simulink model "Syr_ctrl_SFun"  (R2019b)
settings: Solver=ode3  StartTime=0.0  StopTime=0.3  FixedStep=Tstep  MaxStep=1e-5  RelTol=1e-3  AbsTol=1e-3  EnableMultiTasking=on
InitFcn:
  | tic
  | init_sim
  | mex Syr_ctrl.c User_functions\Src\*.c
StopFcn:
  | elapsed_time=toc
values from neighbouring files (symbols this model uses):
  accel = 1000    [init_sim.m]
  B = 0    [init_sim.m]
  Ctrl_type = 3    [init_sim.m]
  dT = motorModel.SyreDrive.Converter.dT    [init_sim.m]
  Fd = motorModel.idiq.Fd    [init_sim.m]
  Fd_dqt = motorModel.dqtMapF.dataF.Fd    [init_sim.m]
  Fd_max = max(Fd_dqt,[],'all')    [init_sim.m]
  Fd_min = min(Fd_dqt,[],'all')    [init_sim.m]
  FMapsModel = -1    [init_sim.m]
  Fq = motorModel.idiq.Fq    [init_sim.m]
  Fq_dqt = motorModel.dqtMapF.dataF.Fq    [init_sim.m]
  Fq_max = max(Fq_dqt,[],'all')    [init_sim.m]
  Fq_min = min(Fq_dqt,[],'all')    [init_sim.m]
  Id_dqt = motorModel.dqtMapF.dataF.Id    [init_sim.m]
  Iq_dqt = motorModel.dqtMapF.dataF.Iq    [init_sim.m]
  J = motorModel.data.J    [init_sim.m]
  P = motorModel.data.p    [init_sim.m]
  Rd = motorModel.SyreDrive.Converter.Rd    [init_sim.m]
  Rs = motorModel.data.Rs    [init_sim.m]
  T_dqt = motorModel.dqtMapF.dataF.T    [init_sim.m]
  th_dqt = motorModel.dqtMapF.dataF.th    [init_sim.m]
  Ts = 200e-6    (= 0.0002)    [init_sim.m]
  Tstep = 2e-6    (= 2e-06)    [init_sim.m]
  V0 = motorModel.SyreDrive.Converter.V0    [init_sim.m]
  VDC = motorModel.data.Vdc    [init_sim.m]
undefined symbols (not defined in the file or in its folder): DiscIntNeverNeededParam, sigbuilder_block
libraries: powerlib_meascontrol x1
settings Model: SimulationMode=accelerator  Creator=work  LastModifiedBy=Dario
settings SolverCC: AutoScaleAbsTol=off
settings DataIOCC: FinalStateName=xFinalSim  InitialState=xFinalSim  SaveFormat=Array  SignalLoggingSaveFormat=ModelDataLogs  SaveOutput=off  SignalLogging=off  DSMLogging=off  TimeSaveName=time  SignalLoggingName=sigsOut
settings OptimizationCC: BlockReduction=off  BooleanDataType=off  ExpressionDepthLimit=2147483647  InitFltsAndDblsToZero=on  LifeSpan=inf
settings DebuggingCC: SaveWithParameterizedLinksMsg=none  UnderspecifiedInitializationDetection=Classic  MergeDetectMultiDrivingBlocksExec=none  SignalResolutionControl=TryResolveAllWithWarning  MultiTaskDSMMsg=warning  MultiTaskCondExecSysMsg=none  FcnCallInpInsideContextMsg=warning  StateNameClashWarn=warning  SFUnexpectedBacktrackingDiag=warning  SFNoUnconditionalDefaultTransitionDiag=warning  SFExecutionAtInitializationDiag=none  ArithmeticOperatorsInVariantConditions=warning
settings HardwareCC: ProdBitPerPointer=32  ProdBitPerSizeT=32  ProdBitPerPtrDiffT=32  ProdLargestAtomicFloat=None  ProdIntDivRoundTo=Undefined  ProdEndianess=Unspecified  ProdWordSize=32  ProdHWDeviceType=32-bit Generic  TargetHWDeviceType=32-bit Generic  TargetUnknown=on  ProdEqTarget=off
settings ModelReferenceCC: PropagateSignalLabelsOutOfModel=off
settings SFSimCC: SimUseLocalCustomCode=off  CustomCodeUndefinedFunction=UseInterfaceOnly
settings RTWCC: RTWUseLocalCustomCode=off
settings CodeAppCC: StateflowObjectComments=on
settings GRTTargetCC: TargetFcnLib=ansi_tfl_tmw.mat  TargetLangStandard=C89/C90 (ANSI)  CombineOutputUpdateFcns=off  GRTInterface=on
settings ConfigComp: CovMetricSettings=dw  CovHtmlReporting=on  CovSaveCumulativeToWorkspaceVar=on  CovSaveSingleToWorkspaceVar=on  CovExternalEMLEnable=off  CovSFcnEnable=off

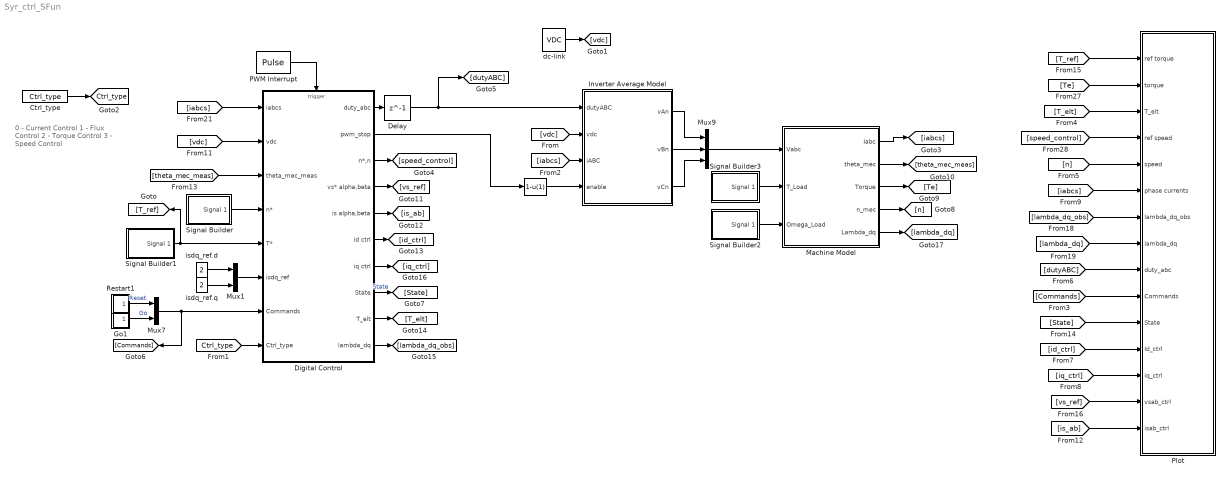
== system Syr_ctrl_SFun ==
  note: 0 - Current Control
      | 1 - Flux Control
      | 2 - Torque Control
      | 3 - Speed Control
  " " : Fcn  Expr=1-u(1)
  Ctrl_type : Constant  Value=Ctrl_type
  Delay : Delay  DelayLength=1
  Digital Control : Subsystem  TreatAsAtomicUnit=on
  Go1 : Subsystem
  Inverter Average Model : Subsystem  mask{TR_mdl=2 Parameters (Von; Rd), TR_par=[0 Rd 3 1.5 0.0714], D_mdl=2 Parameters (Vf; Rd), D_par=[V0 Rd 3 0 0], fsw=1/Ts*1e-3, dead_time=dT*1e6, enable_dt=on, enable_vdrop=on}
      mask prompts: TR_mdl "Choose Transistor model"; TR_par "Transistor parameters [Von1 (V), Rd1 (ohm), Iknee (A), Von2 (V), Rd2 (ohm)]"; D_mdl "Choose Diode model"; D_par "Diode parameters [Vf1 (V), Rd1 (ohm), Iknee (A), Vf2 (V), Rd2 (ohm)]"; fsw "Switching frequency (kHz)"; dead_time "Inverter dead-time (microseconds)"; enable_dt "Enable dead-time effects"; enable_vdrop "Enable on-state voltage drops"
      mask help:
      | This averaged model represents a generic inverter. Select the type of components model to calculate the voltage drop and then insert the parameters value.
      | The requested parameters must be inserted as [von1, Rd1, Iknee, von2 Rd2]. If "2 Parameters" is selected Iknee, von2 and Rd2 are neglected. Iknee is the current at which the voltage drop model passes from (von1, Rd1) to (von2, Rd2).
      mask TypeOptions TR_mdl: 2 Parameters (Von; Rd) | 5 Parameters (Von1; Rd1; Iknee; Von2; Rd2)
      mask TypeOptions D_mdl: 2 Parameters (Vf; Rd) | 5 Parameters (Vf1; Rd1; Iknee; Vf2; Rd2)
      mask Display: plot(0,0,100,100,[39 39 23.8],[71 28 28],[44 56 49.6 56 52.8 56 61 61],[39.2 33.6 32.8 33.6 40.8 33.6 30 12.4],[44 44 44 61 61],[28 71 60 66.4 90],[75 67 83 75 67 83 75 75],[54 42 42 54 54 54 54 66],[61 75 75],[24 24 42],[75 75 61],[66,76,76]);
  Machine Model : Subsystem
  Mux1 : Mux  Inputs=2
  Mux7 : Mux  Inputs=2
  Mux9 : Mux  Inputs=3
  PWM Interrupt : DiscretePulseGenerator  PulseType=Time based  Period=Ts  PulseWidth=50
  Plot : Subsystem
  Restart1 : Subsystem
  Signal Builder : Subsystem  Tag=STV Subsys  LoadFcn=sigbuilder_block('load',[434.4 113.4 550.2 399.6 ]);  StartFcn=sigbuilder_block('start');  StopFcn=sigbuilder_block('stop');  ClipboardFcn=sigbuilder_block('clipboard');  mask(Sigbuilder block){tuvar=[0:10]}
      mask help: Simulink:masks:SigbuilderBlock_MD
      mask init:
      | if ~strcmp(get_param(bdroot(gcbh),'SimulationStatus'),'stopped') tuvar = sigbuilder_block('maskInit'); end
      settings: CopyFcn=sigbuilder_block('copy');  DeleteFcn=sigbuilder_block('delete');  ModelCloseFcn=sigbuilder_block('modelClose');  PreSaveFcn=sigbuilder_block('preSave');  PauseFcn=sigbuilder_block('pause');  ContinueFcn=sigbuilder_block('continue');  NameChangeFcn=sigbuilder_block('namechange');  OpenFcn=sigbuilder_block('open',[434.4 113.4 550.2 399.6 ]);  CloseFcn=sigbuilder_block('close');
      mask Display: plot(0, 0, 100, 100,[2, 2, 32, 32, 2], [68, 8, 8, 68, 68],[32, 2], [38, 38], [32, 19, 2],[53, 60, 44], [32, 17, 17, 2],[16, 16, 31, 31]);txt = getActiveGroup(gcbh);text(2, 100, txt,'verticalAlignment', 'top');
  Signal Builder1 : Subsystem  Tag=STV Subsys  LoadFcn=sigbuilder_block('load');  StartFcn=sigbuilder_block('start');  StopFcn=sigbuilder_block('stop');  ClipboardFcn=sigbuilder_block('clipboard');  mask(Sigbuilder block){tuvar=[0:10]}
      mask help: Simulink:masks:SigbuilderBlock_MD
      mask init:
      | if ~strcmp(get_param(bdroot(gcbh),'SimulationStatus'),'stopped') tuvar = sigbuilder_block('maskInit'); end
      settings: CopyFcn=sigbuilder_block('copy');  DeleteFcn=sigbuilder_block('delete');  ModelCloseFcn=sigbuilder_block('modelClose');  PreSaveFcn=sigbuilder_block('preSave');  PauseFcn=sigbuilder_block('pause');  ContinueFcn=sigbuilder_block('continue');  NameChangeFcn=sigbuilder_block('namechange');  OpenFcn=sigbuilder_block('open',[328.8 83.4 550.2 399.6 ]);  CloseFcn=sigbuilder_block('close');
      mask Display: plot(0, 0, 100, 100,[2, 2, 32, 32, 2], [68, 8, 8, 68, 68],[32, 2], [38, 38], [32, 19, 2],[53, 60, 44], [32, 17, 17, 2],[16, 16, 31, 31]);txt = getActiveGroup(gcbh);text(2, 100, txt,'verticalAlignment', 'top');
  Signal Builder2 : Subsystem  Tag=STV Subsys  LoadFcn=sigbuilder_block('load');  StartFcn=sigbuilder_block('start');  StopFcn=sigbuilder_block('stop');  ClipboardFcn=sigbuilder_block('clipboard');  mask(Sigbuilder block){tuvar=[0:10]}
      mask help: Simulink:masks:SigbuilderBlock_MD
      mask init:
      | if ~strcmp(get_param(bdroot(gcbh),'SimulationStatus'),'stopped') tuvar = sigbuilder_block('maskInit'); end
      settings: CopyFcn=sigbuilder_block('copy');  DeleteFcn=sigbuilder_block('delete');  ModelCloseFcn=sigbuilder_block('modelClose');  PreSaveFcn=sigbuilder_block('preSave');  PauseFcn=sigbuilder_block('pause');  ContinueFcn=sigbuilder_block('continue');  NameChangeFcn=sigbuilder_block('namechange');  OpenFcn=sigbuilder_block('open',[339 112.8 550.2 399.6 ]);  CloseFcn=sigbuilder_block('close');
      mask Display: plot(0, 0, 100, 100,[2, 2, 32, 32, 2], [68, 8, 8, 68, 68],[32, 2], [38, 38], [32, 19, 2],[53, 60, 44], [32, 17, 17, 2],[16, 16, 31, 31]);txt = getActiveGroup(gcbh);text(2, 100, txt,'verticalAlignment', 'top');
  Signal Builder3 : Subsystem  Tag=STV Subsys  LoadFcn=sigbuilder_block('load');  StartFcn=sigbuilder_block('start');  StopFcn=sigbuilder_block('stop');  ClipboardFcn=sigbuilder_block('clipboard');  mask(Sigbuilder block){tuvar=[0:10]}
      mask help: Simulink:masks:SigbuilderBlock_MD
      mask init:
      | if ~strcmp(get_param(bdroot(gcbh),'SimulationStatus'),'stopped') tuvar = sigbuilder_block('maskInit'); end
      settings: CopyFcn=sigbuilder_block('copy');  DeleteFcn=sigbuilder_block('delete');  ModelCloseFcn=sigbuilder_block('modelClose');  PreSaveFcn=sigbuilder_block('preSave');  PauseFcn=sigbuilder_block('pause');  ContinueFcn=sigbuilder_block('continue');  NameChangeFcn=sigbuilder_block('namechange');  OpenFcn=sigbuilder_block('open',[340.5 156 550.5 399.75 ]);  CloseFcn=sigbuilder_block('close');
      mask Display: plot(0, 0, 100, 100,[2, 2, 32, 32, 2], [68, 8, 8, 68, 68],[32, 2], [38, 38], [32, 19, 2],[53, 60, 44], [32, 17, 17, 2],[16, 16, 31, 31]);txt = getActiveGroup(gcbh);text(2, 100, txt,'verticalAlignment', 'top');
  dc-link : Constant  Value=VDC
  isdq_ref.d : Constant  Value=2
  isdq_ref.q : Constant  Value=2
  tag scope: Ctrl_type=global
  wires:
  [iabcs] -> Inverter Average Model/3(iABC)
  dc-link/1 -> [vdc]
  Delay/1 -> [dutyABC], Inverter Average Model/1(dutyABC)
  Digital Control/1(duty_abc) -> Delay/1
  Digital Control/2(pwm_stop) -> " "/1
  [iabcs] -> Digital Control/1(iabcs)
  [vdc] -> Digital Control/2(vdc)
  Mux7/1 -> [Commands], Digital Control/7(Commands)
  Digital Control/3(n*,n) -> [speed_control]
  Digital Control/4(vs* alpha,beta) -> [vs_ref]
  Digital Control/5(is alpha,beta) -> [is_ab]
  Digital Control/6(id ctrl) -> [id_ctrl]
  " "/1 -> Inverter Average Model/4(enable)
  [theta_mec_meas] -> Digital Control/3(theta_mec_meas)
  Digital Control/7(iq ctrl) -> [iq_ctrl]
  PWM Interrupt/1 -> Digital Control/Trigger
  [iabcs] -> Plot/6(phase currents)
  [dutyABC] -> Plot/9(duty_abc)
  Restart1/1(Res) -> Mux7/1  "Reset"
  Go1/1(Go) -> Mux7/2  "Go"
  Signal Builder/1(Signal 1) -> Digital Control/4(n*)
  Machine Model/2(theta_mec) -> [theta_mec_meas]
  Machine Model/1(Iabc) -> [iabcs]
  Mux9/1 -> Machine Model/1(Vabc)
  Signal Builder3/1(Signal 1) -> Machine Model/2(T_Load)
  Inverter Average Model/1(vAn) -> Mux9/1
  Inverter Average Model/2(vBn) -> Mux9/2
  Inverter Average Model/3(vCn) -> Mux9/3
  [vdc] -> Inverter Average Model/2(vdc)
  Mux1/1 -> Digital Control/6(isdq_ref)
  Signal Builder1/1(Signal 1) -> Digital Control/5(T*), [T_ref]
  [Ctrl_type] -> Digital Control/8(Ctrl_type)
  Signal Builder2/1(Signal 1) -> Machine Model/3(Omega_Load)
  isdq_ref.d/1 -> Mux1/1
  isdq_ref.q/1 -> Mux1/2
  [Commands] -> Plot/10(Commands)
  Digital Control/8(State) -> [State]  "State"
  [State] -> Plot/11(State)
  Machine Model/3(Torque) -> [Te]
  Machine Model/4(n_mec) -> [n]
  Digital Control/9(T_elt) -> [T_elt]
  Digital Control/10(lambda_dq) -> [lambda_dq_obs]
  [lambda_dq_obs] -> Plot/7(lambda_dq_obs)
  Machine Model/5(Lambda_dq) -> [lambda_dq]
  [lambda_dq] -> Plot/8(lambda_dq)
  [id_ctrl] -> Plot/12(Id_ctrl)
  [iq_ctrl] -> Plot/13(iq_ctrl)
  [vs_ref] -> Plot/14(vsab_ctrl)
  [is_ab] -> Plot/15(isab_ctrl)
  [T_ref] -> Plot/1(ref torque)
  [Te] -> Plot/2(torque)
  [n] -> Plot/5(speed)
  [speed_control] -> Plot/4(ref speed)
  Ctrl_type/1 -> [Ctrl_type]
  [T_elt] -> Plot/3(T_elt)

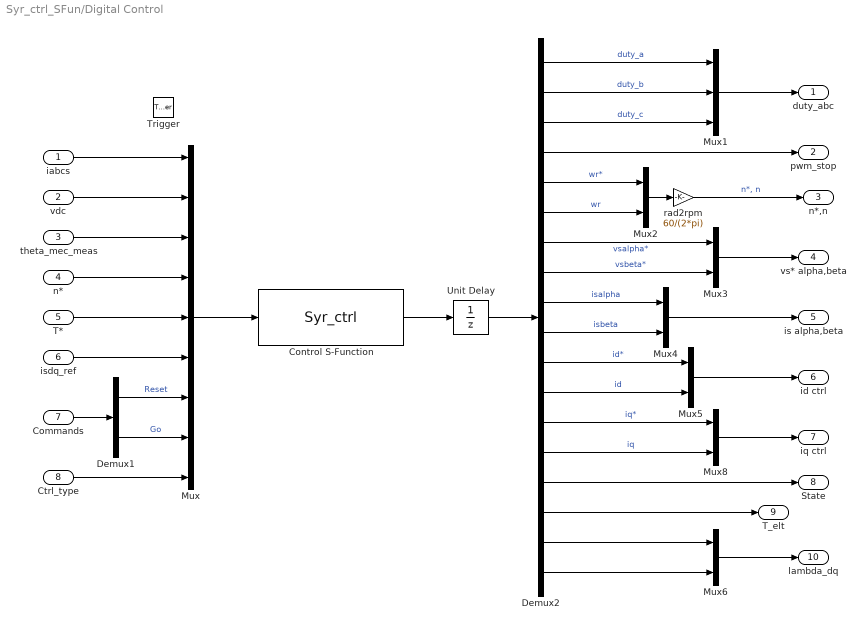
== system Syr_ctrl_SFun/Digital Control ==
  iabcs : Inport
  vdc : Inport  Port=2
  theta_mec_meas : Inport  Port=3
  n* : Inport  Port=4
  T* : Inport  Port=5
  isdq_ref : Inport  Port=6
  Commands : Inport  Port=7
  Ctrl_type : Inport  Port=8
  Trigger : TriggerPort  VariantControl=(inherit)
  Control S-Function : S-Function  FunctionName=Syr_ctrl  SFunctionDeploymentMode=off  EnableBusSupport=off
  Demux1 : Demux  Outputs=2
  Demux2 : Demux  Outputs=18
  Mux : Mux  Inputs=9
  Mux1 : Mux  Inputs=3
  Mux{2..6,8} (6 alike) : Mux  Inputs=2
  Unit Delay : UnitDelay  SampleTime=-1  HasFrameUpgradeWarning=on
  rad2rpm : Gain  Gain=60/(2*pi)
  duty_abc : Outport  VectorParamsAs1DForOutWhenUnconnected=off
  pwm_stop : Outport  Port=2  VectorParamsAs1DForOutWhenUnconnected=off
  n*,n : Outport  Port=3  VectorParamsAs1DForOutWhenUnconnected=off
  vs* alpha,beta : Outport  Port=4  VectorParamsAs1DForOutWhenUnconnected=off
  is alpha,beta : Outport  Port=5  VectorParamsAs1DForOutWhenUnconnected=off
  id ctrl : Outport  Port=6  VectorParamsAs1DForOutWhenUnconnected=off
  iq ctrl : Outport  Port=7  VectorParamsAs1DForOutWhenUnconnected=off
  State : Outport  Port=8  VectorParamsAs1DForOutWhenUnconnected=off
  T_elt : Outport  Port=9  VectorParamsAs1DForOutWhenUnconnected=off
  lambda_dq : Outport  Port=10  VectorParamsAs1DForOutWhenUnconnected=off
  wires:
  Mux/1 -> Control S-Function/1
  iabcs/1 -> Mux/1
  vdc/1 -> Mux/2
  theta_mec_meas/1 -> Mux/3
  Control S-Function/1 -> Unit Delay/1
  Mux4/1 -> is alpha,beta/1
  Mux2/1 -> rad2rpm/1
  Mux3/1 -> vs* alpha,beta/1
  Mux5/1 -> id ctrl/1
  n*/1 -> Mux/4
  rad2rpm/1 -> n*,n/1  "n*, n"
  Mux1/1 -> duty_abc/1
  Mux8/1 -> iq ctrl/1
  Demux1/1 -> Mux/7  "Reset"
  Demux1/2 -> Mux/8  "Go"
  Commands/1 -> Demux1/1
  isdq_ref/1 -> Mux/6
  Unit Delay/1 -> Demux2/1
  Demux2/1 -> Mux1/1  "duty_a"
  Demux2/2 -> Mux1/2  "duty_b"
  Demux2/3 -> Mux1/3  "duty_c"
  Demux2/4 -> pwm_stop/1
  Demux2/15 -> State/1
  T*/1 -> Mux/5
  Ctrl_type/1 -> Mux/9
  Demux2/5 -> Mux2/1  "wr*"
  Demux2/6 -> Mux2/2  "wr"
  Demux2/8 -> Mux3/2  "vsbeta*"
  Demux2/7 -> Mux3/1  "vsalpha*"
  Demux2/9 -> Mux4/1  "isalpha"
  Demux2/10 -> Mux4/2  "isbeta"
  Demux2/12 -> Mux5/2  "id"
  Demux2/11 -> Mux5/1  "id*"
  Demux2/14 -> Mux8/2  "iq"
  Demux2/13 -> Mux8/1  "iq*"
  Demux2/16 -> T_elt/1
  Demux2/17 -> Mux6/1
  Demux2/18 -> Mux6/2
  Mux6/1 -> lambda_dq/1

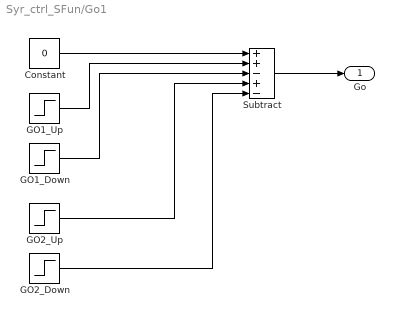
== system Syr_ctrl_SFun/Go1 ==
  Constant : Constant  Value=0
  GO1_Down : Step  Time=0.03+4*Ts  SampleTime=0
  GO1_Up : Step  Time=0.03  SampleTime=0
  GO2_Down : Step  Time=0.1+4*Ts  SampleTime=0
  GO2_Up : Step  Time=0.1  SampleTime=0
  Subtract : Sum  Inputs=++-+-
  Go : Outport  VectorParamsAs1DForOutWhenUnconnected=off
  wires:
  Subtract/1 -> Go/1
  Constant/1 -> Subtract/1
  GO1_Up/1 -> Subtract/2
  GO1_Down/1 -> Subtract/3
  GO2_Up/1 -> Subtract/4
  GO2_Down/1 -> Subtract/5

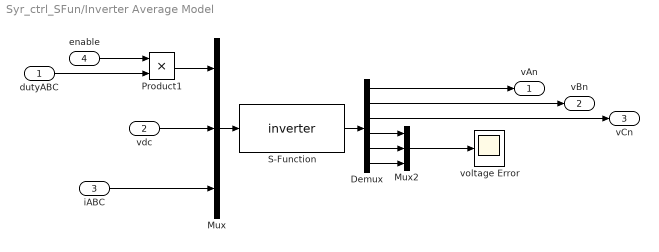
== system Syr_ctrl_SFun/Inverter Average Model ==
  dutyABC : Inport
  vdc : Inport  Port=2
  iABC : Inport  Port=3
  enable : Inport  Port=4
  Demux : Demux  Outputs=6
  Mux : Mux  Inputs=3
  Mux2 : Mux  Inputs=3
  Product1 : Product  RndMeth=Zero
  S-Function : S-Function  FunctionName=inverter  Parameters=fsw,dead_time,enable_dt,enable_vdrop, TR_par(1), TR_par(2), TR_par(3), TR_par(4), TR_par(5), D_par(1), D_par(2), D_par(3), D_par(4), D_par(5), TR_mdl, D_mdl  SFunctionDeploymentMode=off  EnableBusSupport=off
  voltage Error : Scope
  vAn : Outport  VectorParamsAs1DForOutWhenUnconnected=off
  vBn : Outport  Port=2  VectorParamsAs1DForOutWhenUnconnected=off
  vCn : Outport  Port=3  VectorParamsAs1DForOutWhenUnconnected=off
  wires:
  Demux/6 -> Mux2/3
  Demux/5 -> Mux2/2
  Demux/4 -> Mux2/1
  dutyABC/1 -> Product1/2
  Product1/1 -> Mux/1
  Demux/3 -> vCn/1
  Demux/2 -> vBn/1
  Demux/1 -> vAn/1
  iABC/1 -> Mux/3
  vdc/1 -> Mux/2
  Mux/1 -> S-Function/1
  S-Function/1 -> Demux/1
  enable/1 -> Product1/1
  Mux2/1 -> voltage Error/1

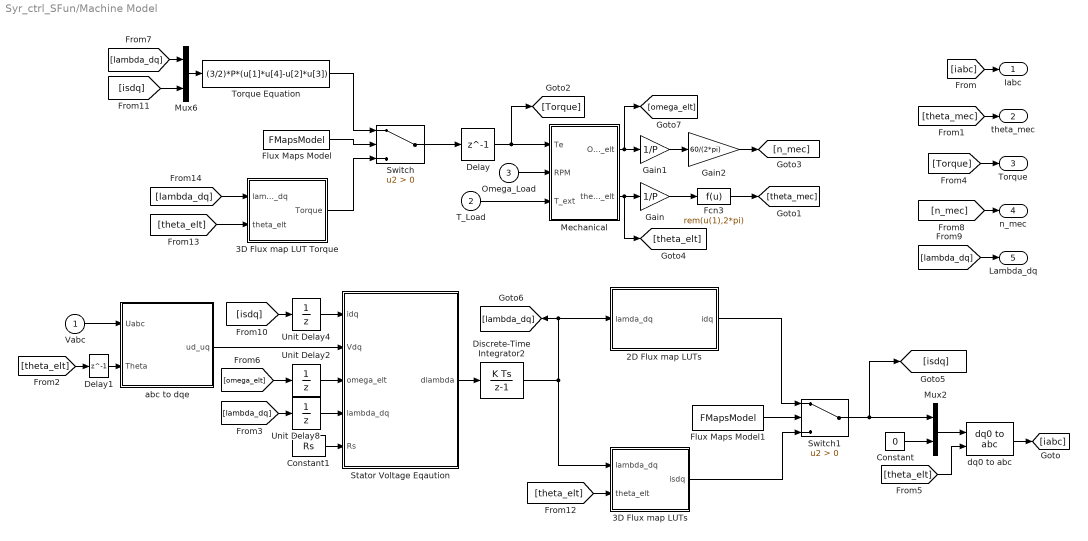
== system Syr_ctrl_SFun/Machine Model ==
  Vabc : Inport
  T_Load : Inport  Port=2
  Omega_Load : Inport  Port=3
  2D Flux map LUTs : Subsystem
  3D Flux map LUT Torque : Subsystem
  3D Flux map LUTs : Subsystem
  Constant : Constant  Value=0
  Constant1 : Constant  Value=Rs
  Delay : Delay  DelayLength=1
  Delay1 : Delay  DelayLength=1  InitialCondition=0
  Discrete-Time Integrator2 : DiscreteIntegrator  gainval=1  SampleTime=Tstep  ICPrevOutput=DiscIntNeverNeededParam  ICPrevScaledInput=DiscIntNeverNeededParam
  Fcn3 : Fcn  Expr=rem(u(1),2*pi)
  Flux Maps Model : Constant  Value=FMapsModel
  Flux Maps Model1 : Constant  Value=FMapsModel
  Gain : Gain  Gain=1/P
  Gain1 : Gain  Gain=1/P
  Gain2 : Gain  Gain=60/(2*pi)
  Mechanical : Subsystem
  Mux2 : Mux  Inputs=2
  Mux6 : Mux  Inputs=2
  Stator Voltage Eqaution : MATLAB Function  TreatAsAtomicUnit=on
  Switch : Switch  Criteria=u2 > Threshold
  Switch1 : Switch  Criteria=u2 > Threshold
  Torque Equation : Fcn  Expr=(3/2)*P*(u[1]*u[4]-u[2]*u[3])
  Unit Delay2 : UnitDelay  SampleTime=-1  HasFrameUpgradeWarning=on
  Unit Delay4 : UnitDelay  SampleTime=-1  HasFrameUpgradeWarning=on
  Unit Delay8 : UnitDelay  SampleTime=-1  HasFrameUpgradeWarning=on
  abc to dqe : Subsystem
  dq0 to abc : powerlib_meascontrol/Transformations/dq0 to abc  Alignment=Aligned with phase A axis
  Iabc : Outport  VectorParamsAs1DForOutWhenUnconnected=off
  theta_mec : Outport  Port=2  VectorParamsAs1DForOutWhenUnconnected=off
  Torque : Outport  Port=3  VectorParamsAs1DForOutWhenUnconnected=off
  n_mec : Outport  Port=4  VectorParamsAs1DForOutWhenUnconnected=off
  Lambda_dq : Outport  Port=5  VectorParamsAs1DForOutWhenUnconnected=off
  wires:
  Fcn3/1 -> [theta_mec]
  Gain/1 -> Fcn3/1
  [isdq] -> Mux6/2
  [isdq] -> Unit Delay4/1
  Unit Delay4/1 -> Stator Voltage Eqaution/1(idq)
  abc to dqe/1(ud_uq) -> Stator Voltage Eqaution/2(Vdq)
  Unit Delay2/1 -> Stator Voltage Eqaution/3(omega_elt)
  [omega_elt] -> Unit Delay2/1
  Constant1/1 -> Stator Voltage Eqaution/5(Rs)
  Unit Delay8/1 -> Stator Voltage Eqaution/4(lambda_dq)
  [lambda_dq] -> Unit Delay8/1
  [lambda_dq] -> Mux6/1
  T_Load/1 -> Mechanical/3(T_ext)
  [theta_elt] -> Delay1/1
  Vabc/1 -> abc to dqe/1(Uabc)
  Mux6/1 -> Torque Equation/1
  Stator Voltage Eqaution/1(dlambda) -> Discrete-Time Integrator2/1
  dq0 to abc/1 -> [iabc]
  Mux2/1 -> dq0 to abc/1
  Constant/1 -> Mux2/2
  [theta_elt] -> dq0 to abc/2
  Mechanical/2(theta_elt) -> [theta_elt], Gain/1
  Omega_Load/1 -> Mechanical/2(RPM)
  [iabc] -> Iabc/1
  [theta_mec] -> theta_mec/1
  [Torque] -> Torque/1
  [n_mec] -> n_mec/1
  [lambda_dq] -> Lambda_dq/1
  Gain1/1 -> Gain2/1
  Gain2/1 -> [n_mec]
  Mechanical/1(Omega_elt) -> [omega_elt], Gain1/1
  Delay1/1 -> abc to dqe/2(Theta)
  Delay/1 -> [Torque], Mechanical/1(Te)
  Switch1/1 -> [isdq], Mux2/1
  [theta_elt] -> 3D Flux map LUTs/2(theta_elt)
  [theta_elt] -> 3D Flux map LUT Torque/2(theta_elt)
  [lambda_dq] -> 3D Flux map LUT Torque/1(" lambda_dq")
  Switch/1 -> Delay/1
  Torque Equation/1 -> Switch/1
  3D Flux map LUT Torque/1(Torque) -> Switch/3
  3D Flux map LUTs/1(isdq) -> Switch1/3
  2D Flux map LUTs/1(idq) -> Switch1/1
  Discrete-Time Integrator2/1 -> 2D Flux map LUTs/1(lamda_dq), [lambda_dq], 3D Flux map LUTs/1(" lambda_dq")
  Flux Maps Model/1 -> Switch/2
  Flux Maps Model1/1 -> Switch1/2

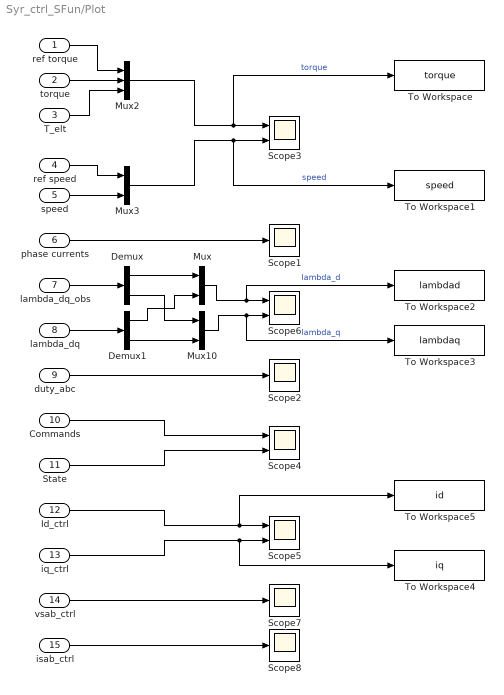
== system Syr_ctrl_SFun/Plot ==
  ref torque : Inport
  torque : Inport  Port=2
  T_elt : Inport  Port=3
  ref speed : Inport  Port=4
  speed : Inport  Port=5
  phase currents : Inport  Port=6
  lambda_dq_obs : Inport  Port=7
  lambda_dq : Inport  Port=8
  duty_abc : Inport  Port=9
  Commands : Inport  Port=10
  State : Inport  Port=11
  Id_ctrl : Inport  Port=12
  iq_ctrl : Inport  Port=13
  vsab_ctrl : Inport  Port=14
  isab_ctrl : Inport  Port=15
  Demux : Demux  Outputs=2
  Demux1 : Demux  Outputs=2
  Mux : Mux  Inputs=2
  Mux10 : Mux  Inputs=2
  Mux2 : Mux  Inputs=3
  Mux3 : Mux  Inputs=2
  Scope{1..2,7..8} (4 alike) : Scope
  Scope{3..6} (4 alike) : Scope  NumInputPorts=2
  To Workspace : ToWorkspace  VariableName=torque  SampleTime=-1
  To Workspace1 : ToWorkspace  VariableName=speed  SampleTime=-1
  To Workspace2 : ToWorkspace  VariableName=lambdad  SampleTime=-1
  To Workspace3 : ToWorkspace  VariableName=lambdaq  SampleTime=-1
  To Workspace4 : ToWorkspace  VariableName=iq  SampleTime=-1
  To Workspace5 : ToWorkspace  VariableName=id  SampleTime=-1
  wires:
  Mux3/1 -> Scope3/2, To Workspace1/1  "speed"
  ref speed/1 -> Mux3/1
  speed/1 -> Mux3/2
  phase currents/1 -> Scope1/1
  Demux/2 -> Mux10/1
  Mux10/1 -> To Workspace3/1, Scope6/2  "lambda_q"
  Demux1/2 -> Mux10/2
  Demux1/1 -> Mux/2
  Demux/1 -> Mux/1
  Mux/1 -> Scope6/1, To Workspace2/1  "lambda_d"
  lambda_dq_obs/1 -> Demux/1
  lambda_dq/1 -> Demux1/1
  duty_abc/1 -> Scope2/1
  Commands/1 -> Scope4/1
  State/1 -> Scope4/2
  T_elt/1 -> Mux2/3
  Id_ctrl/1 -> To Workspace5/1, Scope5/1
  iq_ctrl/1 -> To Workspace4/1, Scope5/2
  vsab_ctrl/1 -> Scope7/1
  isab_ctrl/1 -> Scope8/1
  ref torque/1 -> Mux2/1
  torque/1 -> Mux2/2
  Mux2/1 -> To Workspace/1, Scope3/1  "torque"

== system Syr_ctrl_SFun/Restart1 ==
  "DOWN " : Step  Time=10e-3+4*Ts  SampleTime=0
  Subtract : Sum  Inputs=+-
  "UP " : Step  Time=10e-3  SampleTime=0
  Res : Outport  VectorParamsAs1DForOutWhenUnconnected=off
  wires:
  "UP "/1 -> Subtract/1
  "DOWN "/1 -> Subtract/2
  Subtract/1 -> Res/1

== system Syr_ctrl_SFun/Signal Builder ==
  Demux : Demux  Tag=STV Demux  Outputs=1
  FromWs : FromWorkspace  Tag=STV FromWs  VariableName=tuvar  SampleTime=0
      SigBuilderData=|
      | common.afterFinalStr = 'Extrapolate'
      | common.sampleTime = 0
      | dataSet.timeRange = [0 10]
      | dataSet.name = 'Group 1'
      | sbobj.Groups.Name = 'Group 1'
      | sbobj.Groups.Signals.Name = 'Signal 1'
      | sbobj.Groups.Signals.XData = [0 0.2 1 1 10]
      | sbobj.Groups.Signals.YData = [500 500 500 750 750]
  Signal 1 : Outport  Tag=STV Outport  VectorParamsAs1DForOutWhenUnconnected=off
  wires:
  Demux/1 -> Signal 1/1
  FromWs/1 -> Demux/1

== system Syr_ctrl_SFun/Signal Builder1 ==
  Demux : Demux  Tag=STV Demux  Outputs=1
  FromWs : FromWorkspace  Tag=STV FromWs  VariableName=tuvar  SampleTime=0
      SigBuilderData=|
      | common.afterFinalStr = 'Extrapolate'
      | common.sampleTime = 0
      | dataSet.timeRange = [0 10]
      | dataSet.name = 'Group 1'
      | sbobj.Groups.Name = 'Group 1'
      | sbobj.Groups.Signals.Name = 'Signal 1'
      | sbobj.Groups.Signals.XData = [0 0.125 0.125 5 5 10]
      | sbobj.Groups.Signals.YData = [0 0 7 7 0 0]
  Signal 1 : Outport  Tag=STV Outport  VectorParamsAs1DForOutWhenUnconnected=off
  wires:
  FromWs/1 -> Demux/1
  Demux/1 -> Signal 1/1

== system Syr_ctrl_SFun/Signal Builder2 ==
  Demux : Demux  Tag=STV Demux  Outputs=1
  FromWs : FromWorkspace  Tag=STV FromWs  VariableName=tuvar  SampleTime=0
      SigBuilderData=|
      | common.afterFinalStr = 'Extrapolate'
      | common.sampleTime = 0
      | dataSet.timeRange = [0 10]
      | dataSet.name = 'Group 1'
      | sbobj.Groups.Name = 'Group 1'
      | sbobj.Groups.Signals.Name = 'Signal 1'
      | sbobj.Groups.Signals.XData = [0 0.35 2.5 2.5 10]
      | sbobj.Groups.Signals.YData = [500 500 500 750 750]
  Signal 1 : Outport  Tag=STV Outport  VectorParamsAs1DForOutWhenUnconnected=off
  wires:
  FromWs/1 -> Demux/1
  Demux/1 -> Signal 1/1

== system Syr_ctrl_SFun/Signal Builder3 ==
  Demux : Demux  Tag=STV Demux  Outputs=1
  FromWs : FromWorkspace  Tag=STV FromWs  VariableName=tuvar  SampleTime=0
      SigBuilderData=|
      | common.afterFinalStr = 'Extrapolate'
      | common.sampleTime = 0
      | dataSet.timeRange = [0 10]
      | dataSet.name = 'Group 1'
      | sbobj.Groups.Name = 'Group 1'
      | sbobj.Groups.Signals.Name = 'Signal 1'
      | sbobj.Groups.Signals.XData = [0 1.5 1.5 5 5 10]
      | sbobj.Groups.Signals.YData = [0 0 4 4 0 0]
  Signal 1 : Outport  Tag=STV Outport  VectorParamsAs1DForOutWhenUnconnected=off
  wires:
  Demux/1 -> Signal 1/1
  FromWs/1 -> Demux/1

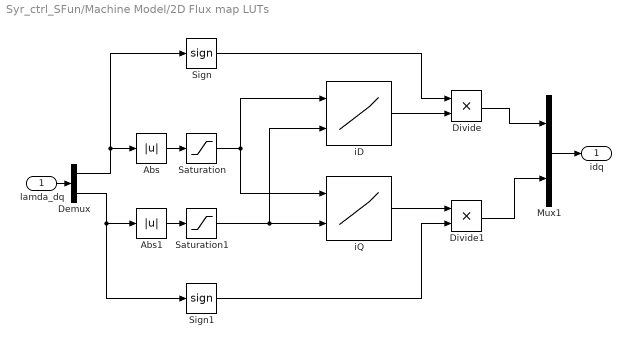
== system Syr_ctrl_SFun/Machine Model/2D Flux map LUTs ==
  lamda_dq : Inport
  Abs : Abs
  Abs1 : Abs
  Demux : Demux  Outputs=2
  Divide : Product  Inputs=**
  Divide1 : Product  Inputs=**
  Mux1 : Mux  Inputs=2
  Saturation : Saturate  UpperLimit=max(max(Fd))  LowerLimit=min(min(Fd))  LinearizeAsGain=off
  Saturation1 : Saturate  UpperLimit=max(max(Fq))  LowerLimit=min(min(Fq))  LinearizeAsGain=off
  Sign : Signum
  Sign1 : Signum
  iD : Lookup_n-D  BreakpointsForDimension1=Fd(1,:)  BreakpointsForDimension2=Fq(:,1)  BreakpointsForDimension1FirstPoint=0  BreakpointsForDimension2FirstPoint=0  BreakpointsForDimension1Spacing=0.17  BreakpointsForDimension2Spacing=0.17  Table=Id'  InternalRulePriority=Speed  RndMeth=Simplest  InputSameDT=on
  iQ : Lookup_n-D  BreakpointsForDimension1=Fd(1,:)  BreakpointsForDimension2=Fq(:,1)  BreakpointsForDimension1FirstPoint=0  BreakpointsForDimension2FirstPoint=0  BreakpointsForDimension1Spacing=0.17  BreakpointsForDimension2Spacing=0.17  Table=Iq'  InternalRulePriority=Speed  RndMeth=Simplest  InputSameDT=on
  idq : Outport  VectorParamsAs1DForOutWhenUnconnected=off
  wires:
  Saturation1/1 -> iQ/2, iD/2
  lamda_dq/1 -> Demux/1
  Divide/1 -> Mux1/1
  iD/1 -> Divide/2
  Sign/1 -> Divide/1
  Mux1/1 -> idq/1
  Saturation/1 -> iQ/1, iD/1
  Demux/2 -> Sign1/1, Abs1/1
  Abs/1 -> Saturation/1
  Demux/1 -> Abs/1, Sign/1
  Abs1/1 -> Saturation1/1
  Divide1/1 -> Mux1/2
  iQ/1 -> Divide1/1
  Sign1/1 -> Divide1/2

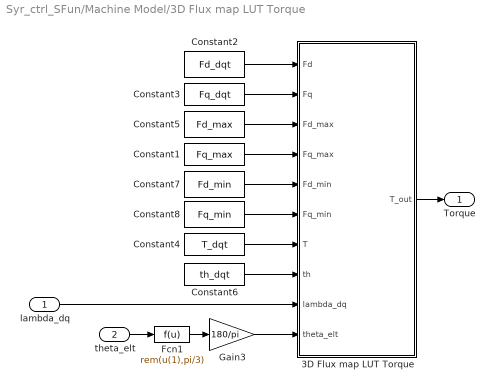
== system Syr_ctrl_SFun/Machine Model/3D Flux map LUT Torque ==
  " lambda_dq" : Inport
  theta_elt : Inport  Port=2
  3D Flux map LUT Torque : MATLAB Function  TreatAsAtomicUnit=on
  Constant1 : Constant  Value=Fq_max
  Constant2 : Constant  Value=Fd_dqt
  Constant3 : Constant  Value=Fq_dqt
  Constant4 : Constant  Value=T_dqt
  Constant5 : Constant  Value=Fd_max
  Constant6 : Constant  Value=th_dqt
  Constant7 : Constant  Value=Fd_min
  Constant8 : Constant  Value=Fq_min
  Fcn1 : Fcn  Expr=rem(u(1),pi/3)
  Gain3 : Gain  Gain=180/pi
  Torque : Outport
  wires:
  3D Flux map LUT Torque/1(T_out) -> Torque/1
  Gain3/1 -> 3D Flux map LUT Torque/10(theta_elt)
  Constant4/1 -> 3D Flux map LUT Torque/7(T)
  Fcn1/1 -> Gain3/1
  Constant2/1 -> 3D Flux map LUT Torque/1(Fd)
  Constant3/1 -> 3D Flux map LUT Torque/2(Fq)
  Constant6/1 -> 3D Flux map LUT Torque/8(th)
  " lambda_dq"/1 -> 3D Flux map LUT Torque/9(lambda_dq)
  theta_elt/1 -> Fcn1/1
  Constant1/1 -> 3D Flux map LUT Torque/4(Fq_max)
  Constant5/1 -> 3D Flux map LUT Torque/3(Fd_max)
  Constant7/1 -> 3D Flux map LUT Torque/5(Fd_min)
  Constant8/1 -> 3D Flux map LUT Torque/6(Fq_min)

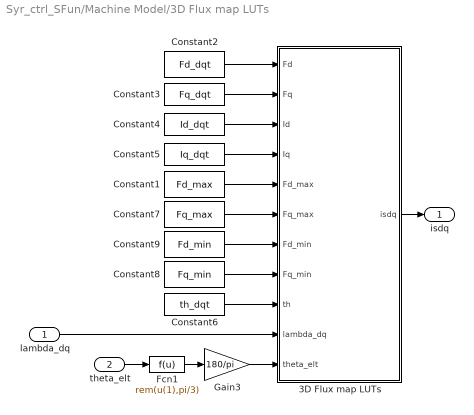
== system Syr_ctrl_SFun/Machine Model/3D Flux map LUTs ==
  " lambda_dq" : Inport
  theta_elt : Inport  Port=2
  3D Flux map LUTs : MATLAB Function  TreatAsAtomicUnit=on
  Constant1 : Constant  Value=Fd_max
  Constant2 : Constant  Value=Fd_dqt
  Constant3 : Constant  Value=Fq_dqt
  Constant4 : Constant  Value=Id_dqt
  Constant5 : Constant  Value=Iq_dqt
  Constant6 : Constant  Value=th_dqt
  Constant7 : Constant  Value=Fq_max
  Constant8 : Constant  Value=Fq_min
  Constant9 : Constant  Value=Fd_min
  Fcn1 : Fcn  Expr=rem(u(1),pi/3)
  Gain3 : Gain  Gain=180/pi
  isdq : Outport
  wires:
  theta_elt/1 -> Fcn1/1
  " lambda_dq"/1 -> 3D Flux map LUTs/10(lambda_dq)
  Constant6/1 -> 3D Flux map LUTs/9(th)
  Constant3/1 -> 3D Flux map LUTs/2(Fq)
  Constant2/1 -> 3D Flux map LUTs/1(Fd)
  Fcn1/1 -> Gain3/1
  Constant4/1 -> 3D Flux map LUTs/3(Id)
  Constant5/1 -> 3D Flux map LUTs/4(Iq)
  Gain3/1 -> 3D Flux map LUTs/11(theta_elt)
  3D Flux map LUTs/1(isdq) -> isdq/1
  Constant1/1 -> 3D Flux map LUTs/5(Fd_max)
  Constant7/1 -> 3D Flux map LUTs/6(Fq_max)
  Constant8/1 -> 3D Flux map LUTs/8(Fq_min)
  Constant9/1 -> 3D Flux map LUTs/7(Fd_min)

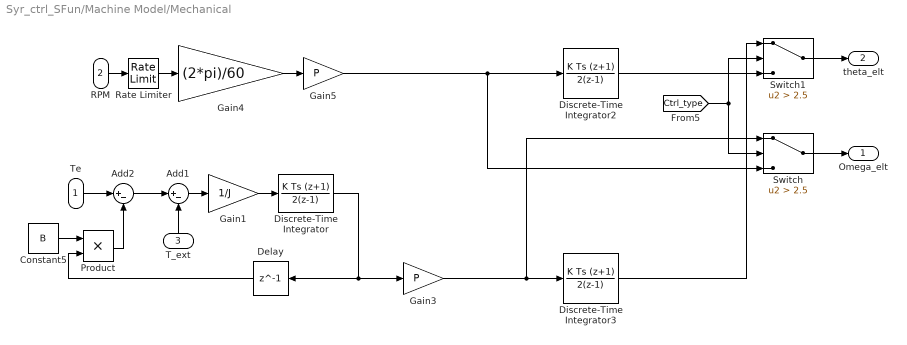
== system Syr_ctrl_SFun/Machine Model/Mechanical ==
  Te : Inport
  RPM : Inport  Port=2
  T_ext : Inport  Port=3
  Add1 : Sum  Inputs=|+-
  Add2 : Sum  Inputs=|+-
  Constant5 : Constant  Value=B
  Delay : Delay  DelayLength=1  InitialCondition=0
  Discrete-Time Integrator : DiscreteIntegrator  IntegratorMethod=Integration: Trapezoidal  gainval=1  SampleTime=Tstep  ICPrevOutput=DiscIntNeverNeededParam  ICPrevScaledInput=DiscIntNeverNeededParam
  Discrete-Time Integrator2 : DiscreteIntegrator  IntegratorMethod=Integration: Trapezoidal  SampleTime=Tstep  ICPrevOutput=DiscIntNeverNeededParam  ICPrevScaledInput=DiscIntNeverNeededParam
  Discrete-Time Integrator3 : DiscreteIntegrator  IntegratorMethod=Integration: Trapezoidal  SampleTime=Tstep  ICPrevOutput=DiscIntNeverNeededParam  ICPrevScaledInput=DiscIntNeverNeededParam
  Gain1 : Gain  Gain=1/J
  Gain3 : Gain  Gain=P
  Gain4 : Gain  Gain=(2*pi)/60
  Gain5 : Gain  Gain=P
  Product : Product
  Rate Limiter : RateLimiter  RisingSlewLimit=accel  FallingSlewLimit=-accel  SampleTimeMode=inherited
  Switch : Switch  Criteria=u2 > Threshold  Threshold=2.5
  Switch1 : Switch  Criteria=u2 > Threshold  Threshold=2.5
  Omega_elt : Outport  VectorParamsAs1DForOutWhenUnconnected=off
  theta_elt : Outport  Port=2  VectorParamsAs1DForOutWhenUnconnected=off
  wires:
  Te/1 -> Add2/1
  Switch/1 -> Omega_elt/1
  Gain3/1 -> Switch/1, Discrete-Time Integrator3/1
  Add2/1 -> Add1/1
  [Ctrl_type] -> Switch/2, Switch1/2
  Discrete-Time Integrator3/1 -> Switch1/1
  Switch1/1 -> theta_elt/1
  Constant5/1 -> Product/1
  Product/1 -> Add2/2
  Gain4/1 -> Gain5/1
  Delay/1 -> Product/2
  Gain5/1 -> Switch/3, Discrete-Time Integrator2/1
  Discrete-Time Integrator2/1 -> Switch1/3
  Add1/1 -> Gain1/1
  Discrete-Time Integrator/1 -> Delay/1, Gain3/1
  Gain1/1 -> Discrete-Time Integrator/1
  T_ext/1 -> Add1/2
  RPM/1 -> Rate Limiter/1
  Rate Limiter/1 -> Gain4/1

== system Syr_ctrl_SFun/Machine Model/abc to dqe ==
  Uabc : Inport
  Theta : Inport  Port=2
  abc to alpabeta : Subsystem
  dqs to dqe : Subsystem
  ud_uq : Outport  VectorParamsAs1DForOutWhenUnconnected=off
  wires:
  dqs to dqe/1(ud_uq) -> ud_uq/1
  Uabc/1 -> abc to alpabeta/1(Uabc)
  Theta/1 -> dqs to dqe/2(Theta)
  abc to alpabeta/1(ualfa_ubeta) -> dqs to dqe/1(ualfa_ubeta)

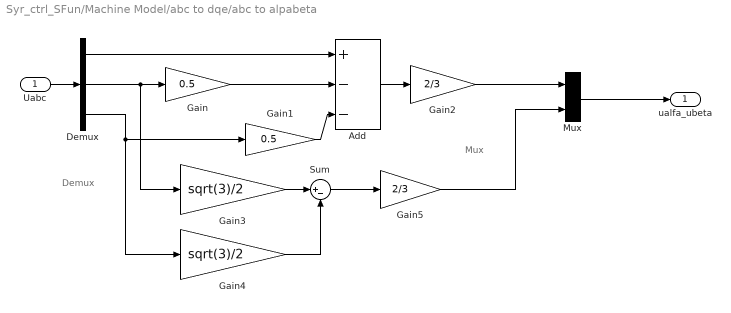
== system Syr_ctrl_SFun/Machine Model/abc to dqe/abc to alpabeta ==
  note: Mux
  note: Demux
  Uabc : Inport
  Add : Sum  Inputs=+--
  Demux : Demux  Outputs=3
  Gain : Gain  Gain=0.5
  Gain1 : Gain  Gain=0.5
  Gain2 : Gain  Gain=2/3
  Gain3 : Gain  Gain=sqrt(3)/2
  Gain4 : Gain  Gain=sqrt(3)/2
  Gain5 : Gain  Gain=2/3
  Mux : Mux  Inputs=2
  Sum : Sum  Inputs=|+-
  ualfa_ubeta : Outport  VectorParamsAs1DForOutWhenUnconnected=off
  wires:
  Uabc/1 -> Demux/1
  Demux/1 -> Add/1
  Demux/2 -> Gain/1, Gain3/1
  Demux/3 -> Gain1/1, Gain4/1
  Gain/1 -> Add/2
  Gain1/1 -> Add/3
  Add/1 -> Gain2/1
  Gain3/1 -> Sum/1
  Gain4/1 -> Sum/2
  Sum/1 -> Gain5/1
  Gain2/1 -> Mux/1
  Gain5/1 -> Mux/2
  Mux/1 -> ualfa_ubeta/1

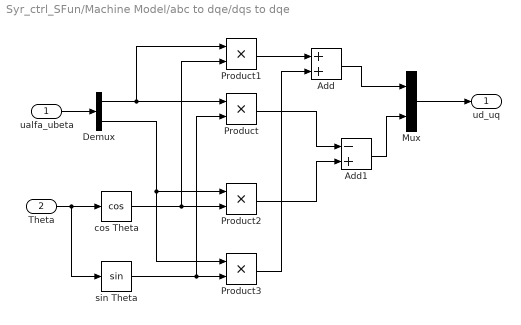
== system Syr_ctrl_SFun/Machine Model/abc to dqe/dqs to dqe ==
  ualfa_ubeta : Inport
  Theta : Inport  Port=2
  Add : Sum
  Add1 : Sum  Inputs=-+
  Demux : Demux  Outputs=2
  Mux : Mux  Inputs=2
  Product{,1..3} (4 alike) : Product  RndMeth=Zero
  cos Theta : Trigonometry  Operator=cos
  sin Theta : Trigonometry
  ud_uq : Outport  VectorParamsAs1DForOutWhenUnconnected=off
  wires:
  ualfa_ubeta/1 -> Demux/1
  Demux/1 -> Product/1, Product1/1
  Theta/1 -> cos Theta/1, sin Theta/1
  cos Theta/1 -> Product2/2, Product1/2
  sin Theta/1 -> Product3/2, Product/2
  Demux/2 -> Product3/1, Product2/1
  Product1/1 -> Add/1
  Product3/1 -> Add/2
  Add/1 -> Mux/1
  Product/1 -> Add1/1
  Product2/1 -> Add1/2
  Add1/1 -> Mux/2
  Mux/1 -> ud_uq/1

== matlab function Syr_ctrl_SFun/Machine Model/3D Flux map LUTs/3D Flux map LUTs ==
  data: Fd input; Fq input; Id input; Iq input; Fd_max input; Fq_max input; Fd_min input; Fq_min input; th input; isdq output; lambda_dq input; theta_elt input
function isdq = fcn(Fd,Fq,Id,Iq,Fd_max,Fq_max,Fd_min,Fq_min,th,lambda_dq,theta_elt)
    isdq = [0; 0];
    
    if theta_elt < min(th,[],'all')
        theta_elt = min(th,[],'all');
    end
    
    sign1 = sign(lambda_dq(1));
    sign2 = sign(lambda_dq(2));

    lambda_dq(1) = abs(lambda_dq(1));
    lambda_dq(2) = abs(lambda_dq(2));
    
    % Flux saturation
    if lambda_dq(1) < Fd_min
        lambda_dq(1) = Fd_min;
    end
    
    if lambda_dq(2) < Fq_min
        lambda_dq(2) = Fq_min;
    end
    
    if lambda_dq(1) > Fd_max
        lambda_dq(1) = Fd_max;
    end
    
    if lambda_dq(2) > Fq_max
        lambda_dq(2) = Fq_max;
    end
   
    % Current interpolation
    isdq(1) = interpn(Fd,Fq,th,Id,lambda_dq(1),lambda_dq(2),theta_elt);
    isdq(2) = interpn(Fd,Fq,th,Iq,lambda_dq(1),lambda_dq(2),theta_elt);
    
    isdq(1) = sign1 * isdq(1);
    isdq(2) = sign2 * isdq(2);
end

== matlab function Syr_ctrl_SFun/Machine Model/Stator Voltage Eqaution ==
  data: idq input; dlambda output; Vdq input; omega_elt input; lambda_dq input; Rs input
function dlambda = fcn(idq, Vdq,omega_elt,lambda_dq, Rs)
dlambda = [0; 0];
dlambda(1) = Vdq(1) - idq(1)*Rs + omega_elt*lambda_dq(2);
dlambda(2) = Vdq(2) - idq(2)*Rs - omega_elt*lambda_dq(1);

== matlab function Syr_ctrl_SFun/Machine Model/3D Flux map LUT Torque/3D Flux map LUT Torque ==
  data: Fd input; Fq input; Fd_max input; Fq_max input; Fd_min input; Fq_min input; T input; th input; T_out output; lambda_dq input; theta_elt input
function T_out = fcn(Fd,Fq,Fd_max,Fq_max,Fd_min,Fq_min,T,th,lambda_dq,theta_elt)
    
    if theta_elt < min(th,[],'all')
        theta_elt = min(th,[],'all');
    end
    
    sign1 = sign(lambda_dq(1));
    sign2 = sign(lambda_dq(2));
    
    lambda_dq(1) = abs(lambda_dq(1));
    lambda_dq(2) = abs(lambda_dq(2));
    
    % Flux saturation 
    if lambda_dq(1) < Fd_min
        lambda_dq(1) = Fd_min;
    end
    
    if lambda_dq(2) < Fq_min
        lambda_dq(2) = Fq_min;
    end
    
    if lambda_dq(1) > Fd_max
        lambda_dq(1) = Fd_max;
    end
    
    if lambda_dq(2) > Fq_max
        lambda_dq(2) = Fq_max;
    end
    
    % Torque interpolation
    T_out = interpn(Fd,Fq,th,T,lambda_dq(1),lambda_dq(2),theta_elt);
    
    T_out = sign1 * sign2 * T_out;

end
